simulink model "Modelo_LTI_equivalente"  (R2017a)
settings: Solver=VariableStepAuto  StartTime=0.0  StopTime=10.0  RelTol=1e-3
values from neighbouring files (symbols this model uses):
  beq = bl/r^2 + bm    (= 1.5638971155e-05)    [Evaluacion_polos_5_2_2.m]    (also in modelo_global_NL.m = 1.5e-05)
  Jeq = Jl/r^2 + Jm    (= 6.9338269301e-06)    [Evaluacion_polos_5_2_2.m]    (also in modelo_global_NL.m = 5.65588462007e-06)
  LambdaM = 0.01546    [Evaluacion_polos_5_2_2.m]    (also in modelo_global_NL.m)
  Lq = 0.0058    [Evaluacion_polos_5_2_2.m]    (also in modelo_global_NL.m)
  Pp = 3    [Evaluacion_polos_5_2_2.m]    (also in modelo_global_NL.m)
  Rs = 1.02    [Evaluacion_polos_5_2_2.m]    (also in modelo_global_NL.m)
settings Model: Creator=merem  LastModifiedBy=merem

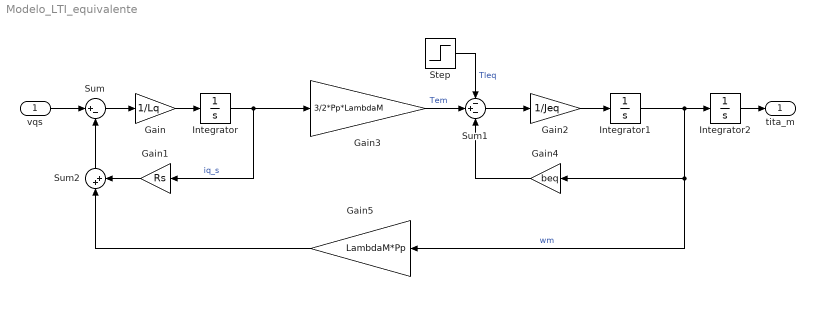
== system Modelo_LTI_equivalente ==
  "vqs " : Inport
  Gain : Gain  Gain=1/Lq
  Gain1 : Gain  Gain=Rs
  Gain2 : Gain  Gain=1/Jeq
  Gain3 : Gain  Gain=3/2*Pp*LambdaM
  Gain4 : Gain  Gain=beq
  Gain5 : Gain  Gain=LambdaM*Pp
  Integrator : Integrator
  Integrator1 : Integrator
  Integrator2 : Integrator
  Step : Step  SampleTime=0
  Sum : Sum  Inputs=|+-
  Sum1 : Sum  Inputs=-+-
  Sum2 : Sum  Inputs=|++
  tita_m : Outport
  wires:
  Sum/1 -> Gain/1
  Gain/1 -> Integrator/1
  Integrator/1 -> Gain1/1, Gain3/1  "iq_s"
  Sum1/1 -> Gain2/1
  Gain2/1 -> Integrator1/1
  Integrator1/1 -> Integrator2/1, Gain5/1, Gain4/1  "wm"
  Gain1/1 -> Sum2/2
  Gain5/1 -> Sum2/1
  Integrator2/1 -> tita_m/1
  Gain4/1 -> Sum1/3
  Gain3/1 -> Sum1/2  "Tem"
  Step/1 -> Sum1/1  "Tleq"
  Sum2/1 -> Sum/2
  "vqs "/1 -> Sum/1
